simulink model "Par2_5_1S"  (R2018a)
settings: Solver=VariableStepAuto  StartTime=0.0  StopTime=6  RelTol=1e-3
settings Model: Creator=wangluo  LastModifiedBy=wangluo

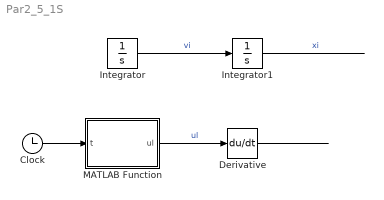
== system Par2_5_1S ==
  Clock : Clock
  Derivative : Derivative
  Integrator : Integrator
  Integrator1 : Integrator
  MATLAB Function : MATLAB Function  TreatAsAtomicUnit=on
  wires:
  Integrator/1 -> Integrator1/1  "vi"
  ? -> Integrator/1  "ui"
  Integrator1/1 -> ?  "xi"
  MATLAB Function/1(ul) -> Derivative/1  "ul"
  Clock/1 -> MATLAB Function/1(t)
  Derivative/1 -> ?

== matlab function Par2_5_1S/MATLAB Function ==
  data: t input; ul output
function ul = fcn(t)

ul = [5 5]' -3 * cos( (t+20)*pi/40 ) * [1 0]'...
                          -3 * sin( (t+20)*pi/40 ) * [0 1]';
% ul = [5 5]' -3 * cos(t) * [1 0]'...
%                           -3 * sin(t) * [0 1]';
